simulink model "toplamaIslemiSimulin"  (R2021b)
settings: Solver=VariableStepAuto  StartTime=0.0  StopTime=20  RelTol=1e-3
values from neighbouring files (symbols this model uses):
  c = 2    [dosya.m]
  f = 5    [dosya.m]
  k = 2    [dosya.m]    (also in durumUzayGosterimi.m = 10)
  m = 1/2    (= 0.5)    [dosya.m]    (also in durumUzayGosterimi.m = 2)
settings Model: Creator=lenovo  LastModifiedBy=lenovo

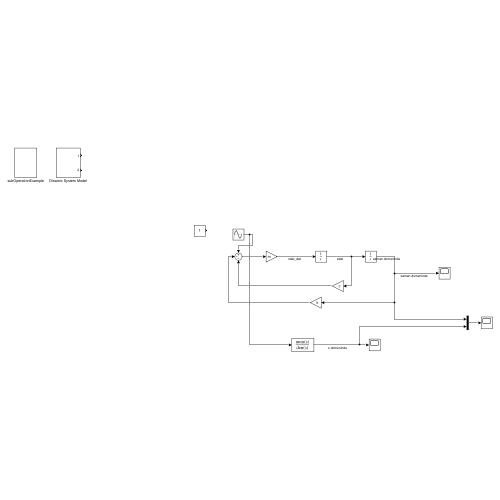
[thumbnail: Simulink's stored preview of the top-level diagram]
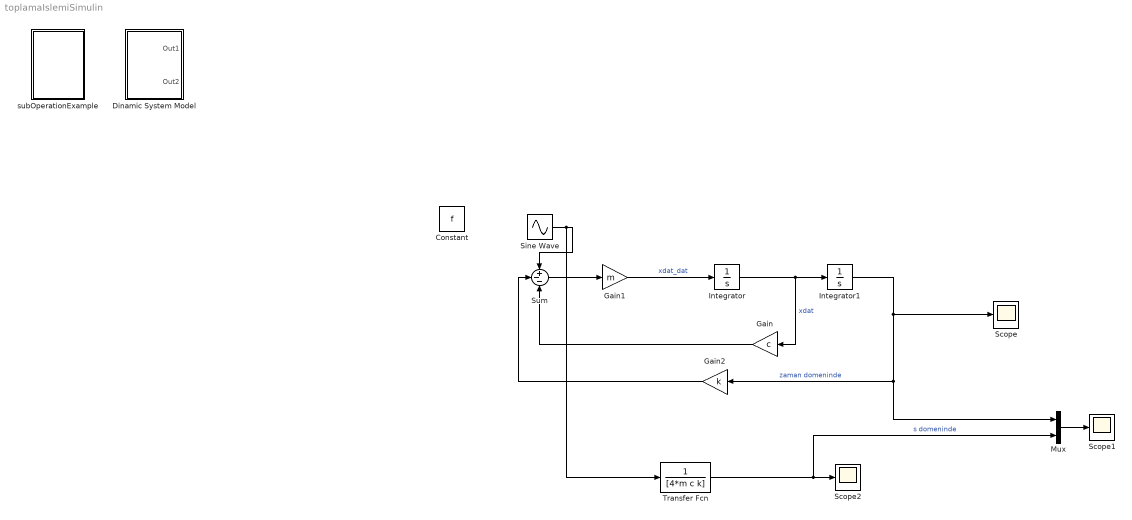
== system toplamaIslemiSimulin ==
  Constant : Constant  Value=f
  Dinamic System Model : Subsystem
  Gain : Gain  Gain=c
  Gain1 : Gain  Gain=m
  Gain2 : Gain  Gain=k
  Integrator : Integrator
  Integrator1 : Integrator
  Mux : Mux  Inputs=2
  Scope : Scope
  Scope1 : Scope
  Scope2 : Scope
  Sine Wave : Sin  Amplitude=5  Bias=5  Frequency=2*pi*1  SampleTime=0
  Sum : Sum  Inputs=+--
  Transfer Fcn : TransferFcn  Denominator=[4*m c k]
  subOperationExample : Subsystem
  wires:
  Gain1/1 -> Integrator/1  "xdat_dat"
  Sum/1 -> Gain1/1
  Gain/1 -> Sum/3
  Integrator/1 -> Gain/1, Integrator1/1  "xdat"
  Integrator1/1 -> Mux/1, Gain2/1, Scope/1  "zaman domeninde"
  Gain2/1 -> Sum/2
  Sine Wave/1 -> Transfer Fcn/1, Sum/1
  Transfer Fcn/1 -> Mux/2, Scope2/1  "s domeninde"
  Mux/1 -> Scope1/1

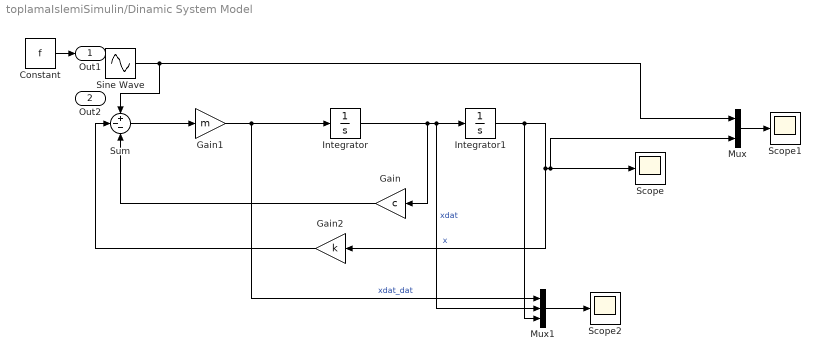
== system toplamaIslemiSimulin/Dinamic System Model ==
  Constant : Constant  Value=f
  Gain : Gain  Gain=c
  Gain1 : Gain  Gain=m
  Gain2 : Gain  Gain=k
  Integrator : Integrator
  Integrator1 : Integrator
  Mux : Mux  Inputs=2
  Mux1 : Mux  Inputs=3
  Scope : Scope
  Scope1 : Scope
  Scope2 : Scope
  Sine Wave : Sin  Amplitude=5  Bias=5  Frequency=2*pi*1  SampleTime=0
  Sum : Sum  Inputs=+--
  Out1 : Outport
  Out2 : Outport  Port=2
  wires:
  Mux1/1 -> Scope2/1
  Gain1/1 -> Mux1/1, Integrator/1  "xdat_dat"
  Sine Wave/1 -> Mux/1, Sum/1
  Gain2/1 -> Sum/2
  Mux/1 -> Scope1/1
  Integrator1/1 -> Mux1/3, Gain2/1, Mux/2, Scope/1  "x"
  Integrator/1 -> Gain/1, Mux1/2, Integrator1/1  "xdat"
  Gain/1 -> Sum/3
  Sum/1 -> Gain1/1
  Constant/1 -> Out1/1

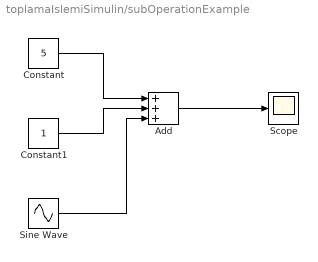
== system toplamaIslemiSimulin/subOperationExample ==
  Add : Sum  Inputs=+++
  Constant : Constant  Value=5
  Constant1 : Constant
  Scope : Scope
  Sine Wave : Sin  Frequency=2*pi*1  SampleTime=0
  wires:
  Constant1/1 -> Add/2
  Add/1 -> Scope/1
  Constant/1 -> Add/1
  Sine Wave/1 -> Add/3
